simulink model "Simpson"  (R2022b)
settings: Solver=FixedStepAuto  StartTime=0.0  StopTime=10.0  RelTol=1e-3
settings Model: Creator=yuzehong  LastModifiedBy=程一帆
settings SolverCC: AlgebraicLoopSolver=TrustRegion
settings OptimizationCC: DefaultParameterBehavior=Inlined  UseDivisionForNetSlopeComputation=on  GainParamInheritBuiltInType=on  UseFloatMulNetSlope=on  InlineInvariantSignals=on  OptimizeBlockIOStorage=off  BufferReuse=off  GlobalBufferReuse=off  ExpressionFolding=off  EnableMemcpy=off  PassReuseOutputArgsAs=Individual arguments  LocalBlockOutputs=off  ZeroExternalMemoryAtStartup=off  ZeroInternalMemoryAtStartup=off  NoFixptDivByZeroProtection=on  EfficientFloat2IntCast=on  LifeSpan=1  OptimizeDataStoreBuffers=off  BusAssignmentInplaceUpdate=off  OptimizationLevel=level0  OptimizationCustomize=off  EfficientTunableParamExpr=on
settings DebuggingCC: ParameterTunabilityLossMsg=error  UnconnectedInputMsg=warning  UnconnectedOutputMsg=warning  UnconnectedLineMsg=warning
settings HardwareCC: ProdLongLongMode=on
settings ModelReferenceCC: EnableRefExpFcnMdlSchedulingChecks=on
settings SFSimCC: MATLABDynamicMemAlloc=off  CustomCodeUndefinedFunction=UseInterfaceOnly
settings RTWCC: Description=Embedded Coder  SystemTargetFile=ert.tlc  TemplateMakefile=ert_default_tmf
settings CodeAppCC: GenerateComments=off  IgnoreCustomStorageClasses=off  OperatorAnnotations=on  SimulinkDataObjDesc=on  SFDataObjDesc=on  CustomSymbolStrGlobalVar=rt$N$M  CustomSymbolStrType=$N$M  CustomSymbolStrFcn=$N$M$F  CustomSymbolStrMacro=$N$M  SimulinkBlockComments=off
settings ERTTargetCC: TargetLangStandard=C99 (ISO)  GenerateSampleERTMain=on  IncludeMdlTerminateFcn=off  CombineSignalStateStructs=on  SupportAbsoluteTime=off  SupportComplex=off  SupportContinuousTime=on  InlinedParameterPlacement=NonHierarchical  ERTCustomFileTemplate=example_file_process.tlc  ERTFilePackagingFormat=CompactWithDataFile

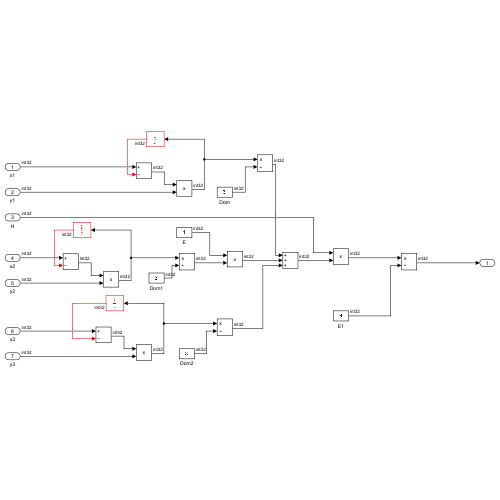
[thumbnail: Simulink's stored preview of the top-level diagram]
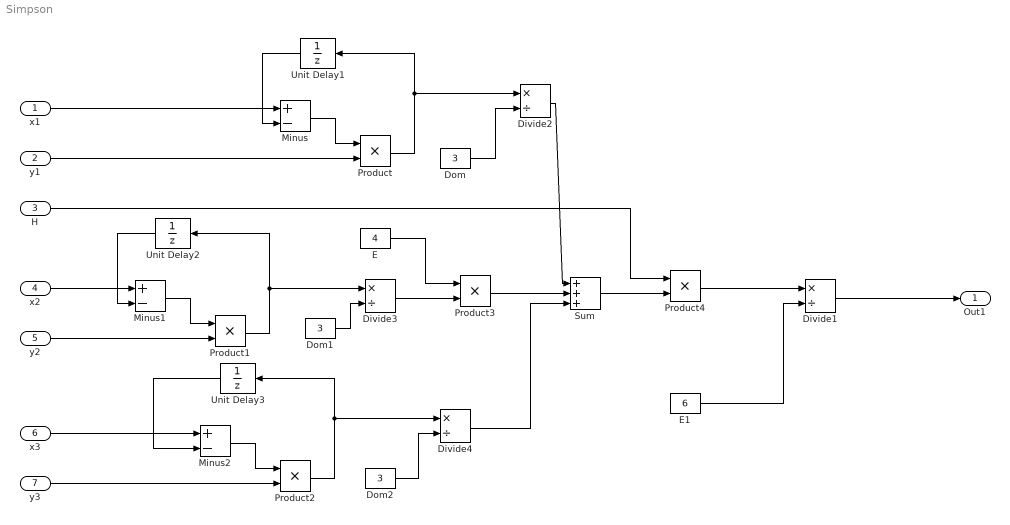
== system Simpson ==
  x1 : Inport  OutDataTypeStr=int32
  y1 : Inport  Port=2  OutDataTypeStr=int32
  H : Inport  Port=3  OutDataTypeStr=int32
  x2 : Inport  Port=4  OutDataTypeStr=int32
  y2 : Inport  Port=5  OutDataTypeStr=int32
  x3 : Inport  Port=6  OutDataTypeStr=int32
  y3 : Inport  Port=7  OutDataTypeStr=int32
  Divide{1..4} (4 alike) : Product  Inputs=*/  OutDataTypeStr=int32
  Dom : Constant  Value=3  OutDataTypeStr=int32
  Dom1 : Constant  Value=3  OutDataTypeStr=int32
  Dom2 : Constant  Value=3  OutDataTypeStr=int32
  E : Constant  Value=4  OutDataTypeStr=int32
  E1 : Constant  Value=6  OutDataTypeStr=int32
  Minus : Sum  Inputs=+-
  Minus1 : Sum  Inputs=+-
  Minus2 : Sum  Inputs=+-
  Product{,1..4} (5 alike) : Product  OutDataTypeStr=int32
  Sum : Sum  Inputs=+++
  Unit Delay1 : UnitDelay  SampleTime=-1  HasFrameUpgradeWarning=on
  Unit Delay2 : UnitDelay  SampleTime=-1  HasFrameUpgradeWarning=on
  Unit Delay3 : UnitDelay  SampleTime=-1  HasFrameUpgradeWarning=on
  Out1 : Outport
  wires:
  x1/1 -> Minus/1
  y1/1 -> Product/2
  Minus/1 -> Product/1
  E/1 -> Product3/1
  Product/1 -> Divide2/1, Unit Delay1/1
  Product3/1 -> Sum/2
  H/1 -> Product4/1
  Sum/1 -> Product4/2
  E1/1 -> Divide1/2
  Divide1/1 -> Out1/1
  Unit Delay1/1 -> Minus/2
  Dom/1 -> Divide2/2
  Divide2/1 -> Sum/1
  Minus1/1 -> Product1/1
  Product1/1 -> Unit Delay2/1, Divide3/1
  Dom1/1 -> Divide3/2
  y2/1 -> Product1/2
  x2/1 -> Minus1/1
  Unit Delay2/1 -> Minus1/2
  Divide3/1 -> Product3/2
  Minus2/1 -> Product2/1
  Product2/1 -> Divide4/1, Unit Delay3/1
  Dom2/1 -> Divide4/2
  y3/1 -> Product2/2
  x3/1 -> Minus2/1
  Unit Delay3/1 -> Minus2/2
  Divide4/1 -> Sum/3
  Product4/1 -> Divide1/1
